simulink model "Swarm_Offline"  (Simulink 8.0)
settings: Solver=ode5  StartTime=0.0  StopTime=inf  FixedStep=sample_time  RelTol=1e-3
InitFcn:
  | sample_time=0.005;%0.004;%0.0025;%0.02;
  | sample_time_Vicon = 0.005;
  | DeltaT = 0.02;
  | g = 9.81;
  | H0 = g%0.3165;
  | Kl = 1;
  | 
  | Q6_mass = 0.73;
  | 
  | Q6_Omega_r = 1.5; %for horizon ref
  | Q6_Zeta_r = 0.5; %for horizon ref
  | Q6_Omega_r_h = 2;%for vertical ref
  | Q6_Zeta_r_h = 1; %for vertical ref
  | 
  | Q6_Omega = 1.5; %for horizon control
  | Q6_Zeta = 0.5; %for horizon control
  | Q6_Omega_h= 2; %for vertical control
  | Q6_Zeta_h = 0.7; %for vertical control
  | 
  | Q6_acc_max = 5;%horizontal max acc
  | Q6_acc_max_h = 3;%horizontal max acc
  | 
  | omega_circle = 36*pi/180;
  | omega_h = 0.1;%Ascending speed
  | PI = pi;
  | Circle_R = 2;
  | MAX_Height = -1;
  | 
  | r0=2; %desired separation distance
  | num = 3; %number of neighbors
  | 
  | load UAV1.mat
  | load UAV2.mat
  | load UAV3.mat
  | load UAV4.mat
libraries: X330_Control x22, simulink x12
(part 2 of 3)

== system Swarm_Offline/Agent 3/Swarming/swarm ==
  agent : Inport
  follower : Inport  Port=2
  2 UAV Swarm Algorithm : MATLAB Function  TreatAsAtomicUnit=on
  Constant : Constant  Value=r0
  agent cmd : Outport
  wires:
  agent/1 -> 2 UAV Swarm Algorithm/1(pos1)
  follower/1 -> 2 UAV Swarm Algorithm/2(pos2)
  2 UAV Swarm Algorithm/2(pos_cmd1) -> agent cmd/1
  Constant/1 -> 2 UAV Swarm Algorithm/3(r0)

== system Swarm_Offline/Agent 3/Swarming/swarm1 ==
  agent : Inport
  follower : Inport  Port=2
  2 UAV Swarm Algorithm : MATLAB Function  TreatAsAtomicUnit=on
  Constant : Constant  Value=r0
  agent cmd : Outport
  wires:
  Constant/1 -> 2 UAV Swarm Algorithm/3(r0)
  2 UAV Swarm Algorithm/2(pos_cmd1) -> agent cmd/1
  follower/1 -> 2 UAV Swarm Algorithm/2(pos2)
  agent/1 -> 2 UAV Swarm Algorithm/1(pos1)

== system Swarm_Offline/Agent 3/Swarming/swarm2 ==
  agent : Inport
  follower : Inport  Port=2
  2 UAV Swarm Algorithm : MATLAB Function  TreatAsAtomicUnit=on
  Constant : Constant  Value=r0
  agent cmd : Outport
  wires:
  agent/1 -> 2 UAV Swarm Algorithm/1(pos1)
  follower/1 -> 2 UAV Swarm Algorithm/2(pos2)
  2 UAV Swarm Algorithm/2(pos_cmd1) -> agent cmd/1
  Constant/1 -> 2 UAV Swarm Algorithm/3(r0)

== system Swarm_Offline/Agent 4/Swarming/swarm ==
  agent : Inport
  follower : Inport  Port=2
  2 UAV Swarm Algorithm : MATLAB Function  TreatAsAtomicUnit=on
  Constant : Constant  Value=r0
  agent cmd : Outport
  wires:
  Constant/1 -> 2 UAV Swarm Algorithm/3(r0)
  2 UAV Swarm Algorithm/2(pos_cmd1) -> agent cmd/1
  follower/1 -> 2 UAV Swarm Algorithm/2(pos2)
  agent/1 -> 2 UAV Swarm Algorithm/1(pos1)

== system Swarm_Offline/Agent 4/Swarming/swarm1 ==
  agent : Inport
  follower : Inport  Port=2
  2 UAV Swarm Algorithm : MATLAB Function  TreatAsAtomicUnit=on
  Constant : Constant  Value=r0
  agent cmd : Outport
  wires:
  agent/1 -> 2 UAV Swarm Algorithm/1(pos1)
  follower/1 -> 2 UAV Swarm Algorithm/2(pos2)
  2 UAV Swarm Algorithm/2(pos_cmd1) -> agent cmd/1
  Constant/1 -> 2 UAV Swarm Algorithm/3(r0)

== system Swarm_Offline/Agent 4/Swarming/swarm2 ==
  agent : Inport
  follower : Inport  Port=2
  2 UAV Swarm Algorithm : MATLAB Function  TreatAsAtomicUnit=on
  Constant : Constant  Value=r0
  agent cmd : Outport
  wires:
  Constant/1 -> 2 UAV Swarm Algorithm/3(r0)
  2 UAV Swarm Algorithm/2(pos_cmd1) -> agent cmd/1
  follower/1 -> 2 UAV Swarm Algorithm/2(pos2)
  agent/1 -> 2 UAV Swarm Algorithm/1(pos1)

== system Swarm_Offline/UAV 1/Trajectory Logic/UAV SF1/Airborne.traj ==
  u : Inport
  f : TriggerPort  TriggerType=function-call
      settings: CopyFcn=Stateflow.SLINSF.SimulinkMan.removeBlockPreDeleteFcn  PreDeleteFcn=Stateflow.SLINSF.SimulinkMan.unsafePredeleteFcn
  Constant : Constant  Value=0
  Enabled Subsystem1 : Subsystem  TreatAsAtomicUnit=on
  Sum : Sum  Inputs=|++
  y1 : Outport
  y2 : Outport  Port=2
  wires:
  Enabled Subsystem1/2(y) -> y2/1
  Enabled Subsystem1/1(x) -> y1/1
  Sum/1 -> Enabled Subsystem1/Enable
  u/1 -> Sum/1
  Constant/1 -> Sum/2

== system Swarm_Offline/UAV 3/Trajectory Logic/UAV SF1/Airborne.traj ==
  u : Inport
  f : TriggerPort  TriggerType=function-call
      settings: CopyFcn=Stateflow.SLINSF.SimulinkMan.removeBlockPreDeleteFcn  PreDeleteFcn=Stateflow.SLINSF.SimulinkMan.unsafePredeleteFcn
  Constant : Constant  Value=0
  Enabled Subsystem1 : Subsystem  TreatAsAtomicUnit=on
  Sum : Sum  Inputs=|++
  y1 : Outport
  y2 : Outport  Port=2
  wires:
  Enabled Subsystem1/2(y) -> y2/1
  Enabled Subsystem1/1(x) -> y1/1
  Sum/1 -> Enabled Subsystem1/Enable
  u/1 -> Sum/1
  Constant/1 -> Sum/2

== system Swarm_Offline/UAV 4/Trajectory Logic/UAV SF1/Airborne.traj ==
  u : Inport
  f : TriggerPort  TriggerType=function-call
      settings: CopyFcn=Stateflow.SLINSF.SimulinkMan.removeBlockPreDeleteFcn  PreDeleteFcn=Stateflow.SLINSF.SimulinkMan.unsafePredeleteFcn
  Constant : Constant  Value=0
  Enabled Subsystem1 : Subsystem  TreatAsAtomicUnit=on
  Sum : Sum  Inputs=|++
  y1 : Outport
  y2 : Outport  Port=2
  wires:
  Constant/1 -> Sum/2
  u/1 -> Sum/1
  Sum/1 -> Enabled Subsystem1/Enable
  Enabled Subsystem1/1(x) -> y1/1
  Enabled Subsystem1/2(y) -> y2/1

== system Swarm_Offline/UAV 5/Trajectory Logic/UAV SF1/Airborne.traj ==
  u : Inport
  f : TriggerPort  TriggerType=function-call
      settings: CopyFcn=Stateflow.SLINSF.SimulinkMan.removeBlockPreDeleteFcn  PreDeleteFcn=Stateflow.SLINSF.SimulinkMan.unsafePredeleteFcn
  Constant : Constant  Value=0
  Enabled Subsystem1 : Subsystem  TreatAsAtomicUnit=on
  Sum : Sum  Inputs=|++
  y1 : Outport
  y2 : Outport  Port=2
  wires:
  Constant/1 -> Sum/2
  u/1 -> Sum/1
  Sum/1 -> Enabled Subsystem1/Enable
  Enabled Subsystem1/1(x) -> y1/1
  Enabled Subsystem1/2(y) -> y2/1

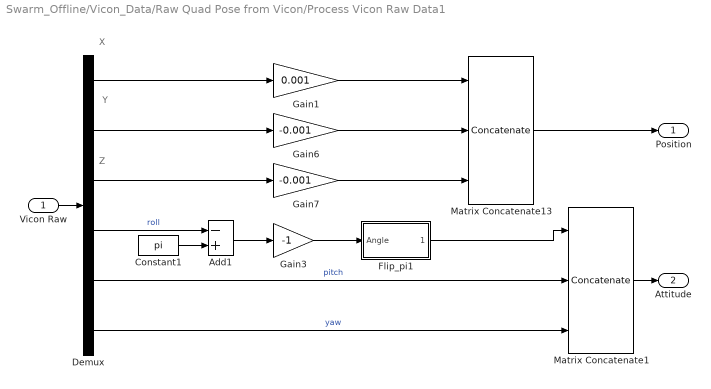
== system Swarm_Offline/Vicon_Data/Raw Quad Pose from Vicon/Process Vicon Raw Data1 ==
  note: X
  note: Y
  note: Z
  Vicon Raw : Inport
  Add1 : Sum  Inputs=-+
  Constant1 : Constant  Value=pi  OutDataTypeStr=double
  Demux : Demux  Outputs=6
  Flip_pi1 : Subsystem  mask(Flip -pi to pi){}
      mask help: Flips the inputs into the range -pi to pi
      mask Help: Flips the inputs into the range -pi to pi
      mask Display: disp('Flip_pi')
  Gain1 : Gain  Gain=0.001
  Gain3 : Gain  Gain=-1
  Gain6 : Gain  Gain=-0.001
  Gain7 : Gain  Gain=-0.001
  Matrix Concatenate1 : Concatenate  NumInputs=3  Mode=Multidimensional array
  Matrix Concatenate13 : Concatenate  NumInputs=3  Mode=Multidimensional array
  Position : Outport
  Attitude : Outport  Port=2
  wires:
  Constant1/1 -> Add1/2
  Demux/6 -> Matrix Concatenate1/3  "yaw"
  Gain1/1 -> Matrix Concatenate13/1
  Demux/1 -> Gain1/1
  Demux/2 -> Gain6/1
  Demux/3 -> Gain7/1
  Demux/4 -> Add1/1  "roll"
  Gain6/1 -> Matrix Concatenate13/2
  Gain7/1 -> Matrix Concatenate13/3
  Add1/1 -> Gain3/1
  Gain3/1 -> Flip_pi1/1(Angle)
  Demux/5 -> Matrix Concatenate1/2  "pitch"
  Flip_pi1/1(Angle_Flip) -> Matrix Concatenate1/1
  Matrix Concatenate13/1 -> Position/1
  Vicon Raw/1 -> Demux/1
  Matrix Concatenate1/1 -> Attitude/1

== system Swarm_Offline/Vicon_Data/Raw Quad Pose from Vicon/Process Vicon Raw Data2 ==
  note: Z
  note: Y
  note: X
  Vicon Raw : Inport
  Add1 : Sum  Inputs=-+
  Constant1 : Constant  Value=pi  OutDataTypeStr=double
  Demux : Demux  Outputs=6
  Flip_pi1 : Subsystem  mask(Flip -pi to pi){}
      mask help: Flips the inputs into the range -pi to pi
      mask Help: Flips the inputs into the range -pi to pi
      mask Display: disp('Flip_pi')
  Gain1 : Gain  Gain=0.001
  Gain3 : Gain  Gain=-1
  Gain6 : Gain  Gain=-0.001
  Gain7 : Gain  Gain=-0.001
  Matrix Concatenate1 : Concatenate  NumInputs=3  Mode=Multidimensional array
  Matrix Concatenate13 : Concatenate  NumInputs=3  Mode=Multidimensional array
  Position : Outport
  Attitude : Outport  Port=2
  wires:
  Matrix Concatenate1/1 -> Attitude/1
  Vicon Raw/1 -> Demux/1
  Matrix Concatenate13/1 -> Position/1
  Flip_pi1/1(Angle_Flip) -> Matrix Concatenate1/1
  Demux/5 -> Matrix Concatenate1/2  "pitch"
  Gain3/1 -> Flip_pi1/1(Angle)
  Add1/1 -> Gain3/1
  Gain7/1 -> Matrix Concatenate13/3
  Gain6/1 -> Matrix Concatenate13/2
  Demux/4 -> Add1/1  "roll"
  Demux/3 -> Gain7/1
  Demux/2 -> Gain6/1
  Demux/1 -> Gain1/1
  Gain1/1 -> Matrix Concatenate13/1
  Demux/6 -> Matrix Concatenate1/3  "yaw"
  Constant1/1 -> Add1/2

== system Swarm_Offline/Vicon_Data/Raw Quad Pose from Vicon/Process Vicon Raw Data3 ==
  note: Z
  note: Y
  note: X
  Vicon Raw : Inport
  Add1 : Sum  Inputs=-+
  Constant1 : Constant  Value=pi  OutDataTypeStr=double
  Demux : Demux  Outputs=6
  Flip_pi1 : Subsystem  mask(Flip -pi to pi){}
      mask help: Flips the inputs into the range -pi to pi
      mask Help: Flips the inputs into the range -pi to pi
      mask Display: disp('Flip_pi')
  Gain1 : Gain  Gain=0.001
  Gain3 : Gain  Gain=-1
  Gain6 : Gain  Gain=-0.001
  Gain7 : Gain  Gain=-0.001
  Matrix Concatenate1 : Concatenate  NumInputs=3  Mode=Multidimensional array
  Matrix Concatenate13 : Concatenate  NumInputs=3  Mode=Multidimensional array
  Position : Outport
  Attitude : Outport  Port=2
  wires:
  Matrix Concatenate1/1 -> Attitude/1
  Vicon Raw/1 -> Demux/1
  Matrix Concatenate13/1 -> Position/1
  Flip_pi1/1(Angle_Flip) -> Matrix Concatenate1/1
  Demux/5 -> Matrix Concatenate1/2  "pitch"
  Gain3/1 -> Flip_pi1/1(Angle)
  Add1/1 -> Gain3/1
  Gain7/1 -> Matrix Concatenate13/3
  Gain6/1 -> Matrix Concatenate13/2
  Demux/4 -> Add1/1  "roll"
  Demux/3 -> Gain7/1
  Demux/2 -> Gain6/1
  Demux/1 -> Gain1/1
  Gain1/1 -> Matrix Concatenate13/1
  Demux/6 -> Matrix Concatenate1/3  "yaw"
  Constant1/1 -> Add1/2

== system Swarm_Offline/Vicon_Data/Raw Quad Pose from Vicon/Process Vicon Raw Data4 ==
  note: X
  note: Y
  note: Z
  Vicon Raw : Inport
  Add1 : Sum  Inputs=-+
  Constant1 : Constant  Value=pi  OutDataTypeStr=double
  Demux : Demux  Outputs=6
  Flip_pi1 : Subsystem  mask(Flip -pi to pi){}
      mask help: Flips the inputs into the range -pi to pi
      mask Help: Flips the inputs into the range -pi to pi
      mask Display: disp('Flip_pi')
  Gain1 : Gain  Gain=0.001
  Gain3 : Gain  Gain=-1
  Gain6 : Gain  Gain=-0.001
  Gain7 : Gain  Gain=-0.001
  Matrix Concatenate1 : Concatenate  NumInputs=3  Mode=Multidimensional array
  Matrix Concatenate13 : Concatenate  NumInputs=3  Mode=Multidimensional array
  Position : Outport
  Attitude : Outport  Port=2
  wires:
  Constant1/1 -> Add1/2
  Demux/6 -> Matrix Concatenate1/3  "yaw"
  Gain1/1 -> Matrix Concatenate13/1
  Demux/1 -> Gain1/1
  Demux/2 -> Gain6/1
  Demux/3 -> Gain7/1
  Demux/4 -> Add1/1  "roll"
  Gain6/1 -> Matrix Concatenate13/2
  Gain7/1 -> Matrix Concatenate13/3
  Add1/1 -> Gain3/1
  Gain3/1 -> Flip_pi1/1(Angle)
  Demux/5 -> Matrix Concatenate1/2  "pitch"
  Flip_pi1/1(Angle_Flip) -> Matrix Concatenate1/1
  Matrix Concatenate13/1 -> Position/1
  Vicon Raw/1 -> Demux/1
  Matrix Concatenate1/1 -> Attitude/1

== system Swarm_Offline/Vicon_Data/Raw Quad Pose from Vicon/Process Vicon Raw Data6 ==
  note: X
  note: Y
  note: Z
  Vicon Raw : Inport
  Add1 : Sum  Inputs=-+
  Constant1 : Constant  Value=pi  OutDataTypeStr=double
  Demux : Demux  Outputs=6
  Flip_pi1 : Subsystem  mask(Flip -pi to pi){}
      mask help: Flips the inputs into the range -pi to pi
      mask Help: Flips the inputs into the range -pi to pi
      mask Display: disp('Flip_pi')
  Gain1 : Gain  Gain=0.001
  Gain3 : Gain  Gain=-1
  Gain6 : Gain  Gain=-0.001
  Gain7 : Gain  Gain=-0.001
  Matrix Concatenate1 : Concatenate  NumInputs=3  Mode=Multidimensional array
  Matrix Concatenate13 : Concatenate  NumInputs=3  Mode=Multidimensional array
  Position : Outport
  Attitude : Outport  Port=2
  wires:
  Constant1/1 -> Add1/2
  Demux/6 -> Matrix Concatenate1/3  "yaw"
  Gain1/1 -> Matrix Concatenate13/1
  Demux/1 -> Gain1/1
  Demux/2 -> Gain6/1
  Demux/3 -> Gain7/1
  Demux/4 -> Add1/1  "roll"
  Gain6/1 -> Matrix Concatenate13/2
  Gain7/1 -> Matrix Concatenate13/3
  Add1/1 -> Gain3/1
  Gain3/1 -> Flip_pi1/1(Angle)
  Demux/5 -> Matrix Concatenate1/2  "pitch"
  Flip_pi1/1(Angle_Flip) -> Matrix Concatenate1/1
  Matrix Concatenate13/1 -> Position/1
  Vicon Raw/1 -> Demux/1
  Matrix Concatenate1/1 -> Attitude/1

== system Swarm_Offline/Vicon_Data/Raw Quad Pose from Vicon/Process Vicon Raw Data7 ==
  note: Z
  note: Y
  note: X
  Vicon Raw : Inport
  Add1 : Sum  Inputs=-+
  Constant1 : Constant  Value=pi  OutDataTypeStr=double
  Demux : Demux  Outputs=6
  Flip_pi1 : Subsystem  mask(Flip -pi to pi){}
      mask help: Flips the inputs into the range -pi to pi
      mask Help: Flips the inputs into the range -pi to pi
      mask Display: disp('Flip_pi')
  Gain1 : Gain  Gain=0.001
  Gain3 : Gain  Gain=-1
  Gain6 : Gain  Gain=-0.001
  Gain7 : Gain  Gain=-0.001
  Matrix Concatenate1 : Concatenate  NumInputs=3  Mode=Multidimensional array
  Matrix Concatenate13 : Concatenate  NumInputs=3  Mode=Multidimensional array
  Position : Outport
  Attitude : Outport  Port=2
  wires:
  Matrix Concatenate1/1 -> Attitude/1
  Vicon Raw/1 -> Demux/1
  Matrix Concatenate13/1 -> Position/1
  Flip_pi1/1(Angle_Flip) -> Matrix Concatenate1/1
  Demux/5 -> Matrix Concatenate1/2  "pitch"
  Gain3/1 -> Flip_pi1/1(Angle)
  Add1/1 -> Gain3/1
  Gain7/1 -> Matrix Concatenate13/3
  Gain6/1 -> Matrix Concatenate13/2
  Demux/4 -> Add1/1  "roll"
  Demux/3 -> Gain7/1
  Demux/2 -> Gain6/1
  Demux/1 -> Gain1/1
  Gain1/1 -> Matrix Concatenate13/1
  Demux/6 -> Matrix Concatenate1/3  "yaw"
  Constant1/1 -> Add1/2

== system Swarm_Offline/UAV 1/Trajectory Logic/UAV SF1/Airborne.traj/Enabled Subsystem1 ==
  Enable : EnablePort
  From Workspace : FromWorkspace  VariableName=UAV1  Interpolate=off  OutputAfterFinalValue=Holding final value
  Selector1 : Selector  InputPortWidth=2  IndexOptions=Index vector (dialog)  Indices=[2]  OutputSizes=1
  Selector6 : Selector  InputPortWidth=2  IndexOptions=Index vector (dialog)  Indices=[1]  OutputSizes=1
  x : Outport
  y : Outport  Port=2
  z : Outport  Port=3
  Psi : Outport  Port=4
  wires:
  Selector1/1 -> y/1
  Selector6/1 -> x/1
  From Workspace/1 -> Selector6/1, Selector1/1

== system Swarm_Offline/UAV 3/Trajectory Logic/UAV SF1/Airborne.traj/Enabled Subsystem1 ==
  Enable : EnablePort
  From Workspace : FromWorkspace  VariableName=UAV2  Interpolate=off  OutputAfterFinalValue=Holding final value
  Selector1 : Selector  InputPortWidth=2  IndexOptions=Index vector (dialog)  Indices=[1]  OutputSizes=1
  Selector6 : Selector  InputPortWidth=2  IndexOptions=Index vector (dialog)  Indices=[1]  OutputSizes=1
  x : Outport
  y : Outport  Port=2
  z : Outport  Port=3
  Psi : Outport  Port=4
  wires:
  Selector6/1 -> y/1
  Selector1/1 -> x/1
  From Workspace/1 -> Selector1/1, Selector6/1

== system Swarm_Offline/UAV 4/Trajectory Logic/UAV SF1/Airborne.traj/Enabled Subsystem1 ==
  Enable : EnablePort
  From Workspace : FromWorkspace  VariableName=UAV3  Interpolate=off  OutputAfterFinalValue=Holding final value
  Selector1 : Selector  InputPortWidth=2  IndexOptions=Index vector (dialog)  Indices=[1]  OutputSizes=1
  Selector6 : Selector  InputPortWidth=2  IndexOptions=Index vector (dialog)  Indices=[1]  OutputSizes=1
  x : Outport
  y : Outport  Port=2
  z : Outport  Port=3
  psi : Outport  Port=4
  wires:
  From Workspace/1 -> Selector1/1, Selector6/1
  Selector1/1 -> x/1
  Selector6/1 -> y/1

== system Swarm_Offline/UAV 5/Trajectory Logic/UAV SF1/Airborne.traj/Enabled Subsystem1 ==
  Enable : EnablePort
  From Workspace : FromWorkspace  VariableName=UAV4  Interpolate=off  OutputAfterFinalValue=Holding final value
  Selector1 : Selector  InputPortWidth=2  IndexOptions=Index vector (dialog)  Indices=[1]  OutputSizes=1
  Selector6 : Selector  InputPortWidth=2  IndexOptions=Index vector (dialog)  Indices=[1]  OutputSizes=1
  x : Outport
  y : Outport  Port=2
  z : Outport  Port=3
  Psi : Outport  Port=4
  wires:
  From Workspace/1 -> Selector6/1, Selector1/1
  Selector1/1 -> x/1
  Selector6/1 -> y/1

== system Swarm_Offline/Vicon_Data/Raw Quad Pose from Vicon/Process Vicon Raw Data1/Flip_pi1 ==
  Angle : Inport
  Add : Sum  Inputs=-+
  Compare To Constant1 : simulink/Logic and Bit Operations/Compare To Constant  relop=>  const=pi  OutDataTypeStr=uint8  ZeroCross=off
  Constant : Constant  Value=2*pi
  Data Type Duplicate : DataTypeDuplicate
  Flip_0_to_2pi : Subsystem  mask(Flip zero to 2pi){}
      mask help: Flips the inputs into the range zero to +2pi
      mask Help: Flips the inputs into the range zero to +2pi
      mask Display: disp('Flip_0_2pi')
  Switch : Switch  Criteria=u2 ~= 0
  Angle_Flip : Outport
  wires:
  Switch/1 -> Data Type Duplicate/1, Angle_Flip/1
  Add/1 -> Switch/1
  Constant/1 -> Add/1
  Compare To Constant1/1 -> Switch/2
  Flip_0_to_2pi/1(Angle_Flip) -> Add/2, Compare To Constant1/1, Switch/3
  Angle/1 -> Data Type Duplicate/2, Flip_0_to_2pi/1(Angle)

== system Swarm_Offline/Vicon_Data/Raw Quad Pose from Vicon/Process Vicon Raw Data2/Flip_pi1 ==
  Angle : Inport
  Add : Sum  Inputs=-+
  Compare To Constant1 : simulink/Logic and Bit Operations/Compare To Constant  relop=>  const=pi  OutDataTypeStr=uint8  ZeroCross=off
  Constant : Constant  Value=2*pi
  Data Type Duplicate : DataTypeDuplicate
  Flip_0_to_2pi : Subsystem  mask(Flip zero to 2pi){}
      mask help: Flips the inputs into the range zero to +2pi
      mask Help: Flips the inputs into the range zero to +2pi
      mask Display: disp('Flip_0_2pi')
  Switch : Switch  Criteria=u2 ~= 0
  Angle_Flip : Outport
  wires:
  Angle/1 -> Flip_0_to_2pi/1(Angle), Data Type Duplicate/2
  Flip_0_to_2pi/1(Angle_Flip) -> Switch/3, Compare To Constant1/1, Add/2
  Compare To Constant1/1 -> Switch/2
  Constant/1 -> Add/1
  Add/1 -> Switch/1
  Switch/1 -> Angle_Flip/1, Data Type Duplicate/1

== system Swarm_Offline/Vicon_Data/Raw Quad Pose from Vicon/Process Vicon Raw Data3/Flip_pi1 ==
  Angle : Inport
  Add : Sum  Inputs=-+
  Compare To Constant1 : simulink/Logic and Bit Operations/Compare To Constant  relop=>  const=pi  OutDataTypeStr=uint8  ZeroCross=off
  Constant : Constant  Value=2*pi
  Data Type Duplicate : DataTypeDuplicate
  Flip_0_to_2pi : Subsystem  mask(Flip zero to 2pi){}
      mask help: Flips the inputs into the range zero to +2pi
      mask Help: Flips the inputs into the range zero to +2pi
      mask Display: disp('Flip_0_2pi')
  Switch : Switch  Criteria=u2 ~= 0
  Angle_Flip : Outport
  wires:
  Angle/1 -> Flip_0_to_2pi/1(Angle), Data Type Duplicate/2
  Flip_0_to_2pi/1(Angle_Flip) -> Switch/3, Compare To Constant1/1, Add/2
  Compare To Constant1/1 -> Switch/2
  Constant/1 -> Add/1
  Add/1 -> Switch/1
  Switch/1 -> Angle_Flip/1, Data Type Duplicate/1

== system Swarm_Offline/Vicon_Data/Raw Quad Pose from Vicon/Process Vicon Raw Data4/Flip_pi1 ==
  Angle : Inport
  Add : Sum  Inputs=-+
  Compare To Constant1 : simulink/Logic and Bit Operations/Compare To Constant  relop=>  const=pi  OutDataTypeStr=uint8  ZeroCross=off
  Constant : Constant  Value=2*pi
  Data Type Duplicate : DataTypeDuplicate
  Flip_0_to_2pi : Subsystem  mask(Flip zero to 2pi){}
      mask help: Flips the inputs into the range zero to +2pi
      mask Help: Flips the inputs into the range zero to +2pi
      mask Display: disp('Flip_0_2pi')
  Switch : Switch  Criteria=u2 ~= 0
  Angle_Flip : Outport
  wires:
  Switch/1 -> Data Type Duplicate/1, Angle_Flip/1
  Add/1 -> Switch/1
  Constant/1 -> Add/1
  Compare To Constant1/1 -> Switch/2
  Flip_0_to_2pi/1(Angle_Flip) -> Add/2, Compare To Constant1/1, Switch/3
  Angle/1 -> Data Type Duplicate/2, Flip_0_to_2pi/1(Angle)

== system Swarm_Offline/Vicon_Data/Raw Quad Pose from Vicon/Process Vicon Raw Data6/Flip_pi1 ==
  Angle : Inport
  Add : Sum  Inputs=-+
  Compare To Constant1 : simulink/Logic and Bit Operations/Compare To Constant  relop=>  const=pi  OutDataTypeStr=uint8  ZeroCross=off
  Constant : Constant  Value=2*pi
  Data Type Duplicate : DataTypeDuplicate
  Flip_0_to_2pi : Subsystem  mask(Flip zero to 2pi){}
      mask help: Flips the inputs into the range zero to +2pi
      mask Help: Flips the inputs into the range zero to +2pi
      mask Display: disp('Flip_0_2pi')
  Switch : Switch  Criteria=u2 ~= 0
  Angle_Flip : Outport
  wires:
  Switch/1 -> Data Type Duplicate/1, Angle_Flip/1
  Add/1 -> Switch/1
  Constant/1 -> Add/1
  Compare To Constant1/1 -> Switch/2
  Flip_0_to_2pi/1(Angle_Flip) -> Add/2, Compare To Constant1/1, Switch/3
  Angle/1 -> Data Type Duplicate/2, Flip_0_to_2pi/1(Angle)

== system Swarm_Offline/Vicon_Data/Raw Quad Pose from Vicon/Process Vicon Raw Data7/Flip_pi1 ==
  Angle : Inport
  Add : Sum  Inputs=-+
  Compare To Constant1 : simulink/Logic and Bit Operations/Compare To Constant  relop=>  const=pi  OutDataTypeStr=uint8  ZeroCross=off
  Constant : Constant  Value=2*pi
  Data Type Duplicate : DataTypeDuplicate
  Flip_0_to_2pi : Subsystem  mask(Flip zero to 2pi){}
      mask help: Flips the inputs into the range zero to +2pi
      mask Help: Flips the inputs into the range zero to +2pi
      mask Display: disp('Flip_0_2pi')
  Switch : Switch  Criteria=u2 ~= 0
  Angle_Flip : Outport
  wires:
  Angle/1 -> Flip_0_to_2pi/1(Angle), Data Type Duplicate/2
  Flip_0_to_2pi/1(Angle_Flip) -> Switch/3, Compare To Constant1/1, Add/2
  Compare To Constant1/1 -> Switch/2
  Constant/1 -> Add/1
  Add/1 -> Switch/1
  Switch/1 -> Angle_Flip/1, Data Type Duplicate/1

== system Swarm_Offline/Vicon_Data/Raw Quad Pose from Vicon/Process Vicon Raw Data1/Flip_pi1/Flip_0_to_2pi ==
  Angle : Inport
  Add : Sum
  Compare To Constant1 : simulink/Logic and Bit Operations/Compare To Constant  relop=<  const=0  OutDataTypeStr=uint8  ZeroCross=off
  Constant : Constant  Value=2*pi
  Data Type Duplicate : DataTypeDuplicate
  Flip_2pi : Subsystem  mask(Flip -2pi to 2pi){}
      mask help: Flips the inputs into the range -2pi to +2pi
      mask Help: Flips the inputs into the range -2pi to +2pi
      mask Display: disp('Flip_2pi')
  Switch : Switch  Criteria=u2 ~= 0
  Angle_Flip : Outport
  wires:
  Switch/1 -> Data Type Duplicate/1, Angle_Flip/1
  Angle/1 -> Data Type Duplicate/2, Flip_2pi/1(Angle)
  Add/1 -> Switch/1
  Constant/1 -> Add/1
  Compare To Constant1/1 -> Switch/2
  Flip_2pi/1(Angle_Flip) -> Switch/3, Add/2, Compare To Constant1/1

== system Swarm_Offline/Vicon_Data/Raw Quad Pose from Vicon/Process Vicon Raw Data2/Flip_pi1/Flip_0_to_2pi ==
  Angle : Inport
  Add : Sum
  Compare To Constant1 : simulink/Logic and Bit Operations/Compare To Constant  relop=<  const=0  OutDataTypeStr=uint8  ZeroCross=off
  Constant : Constant  Value=2*pi
  Data Type Duplicate : DataTypeDuplicate
  Flip_2pi : Subsystem  mask(Flip -2pi to 2pi){}
      mask help: Flips the inputs into the range -2pi to +2pi
      mask Help: Flips the inputs into the range -2pi to +2pi
      mask Display: disp('Flip_2pi')
  Switch : Switch  Criteria=u2 ~= 0
  Angle_Flip : Outport
  wires:
  Flip_2pi/1(Angle_Flip) -> Compare To Constant1/1, Add/2, Switch/3
  Compare To Constant1/1 -> Switch/2
  Constant/1 -> Add/1
  Add/1 -> Switch/1
  Angle/1 -> Flip_2pi/1(Angle), Data Type Duplicate/2
  Switch/1 -> Angle_Flip/1, Data Type Duplicate/1

== system Swarm_Offline/Vicon_Data/Raw Quad Pose from Vicon/Process Vicon Raw Data3/Flip_pi1/Flip_0_to_2pi ==
  Angle : Inport
  Add : Sum
  Compare To Constant1 : simulink/Logic and Bit Operations/Compare To Constant  relop=<  const=0  OutDataTypeStr=uint8  ZeroCross=off
  Constant : Constant  Value=2*pi
  Data Type Duplicate : DataTypeDuplicate
  Flip_2pi : Subsystem  mask(Flip -2pi to 2pi){}
      mask help: Flips the inputs into the range -2pi to +2pi
      mask Help: Flips the inputs into the range -2pi to +2pi
      mask Display: disp('Flip_2pi')
  Switch : Switch  Criteria=u2 ~= 0
  Angle_Flip : Outport
  wires:
  Flip_2pi/1(Angle_Flip) -> Compare To Constant1/1, Add/2, Switch/3
  Compare To Constant1/1 -> Switch/2
  Constant/1 -> Add/1
  Add/1 -> Switch/1
  Angle/1 -> Flip_2pi/1(Angle), Data Type Duplicate/2
  Switch/1 -> Angle_Flip/1, Data Type Duplicate/1

== system Swarm_Offline/Vicon_Data/Raw Quad Pose from Vicon/Process Vicon Raw Data4/Flip_pi1/Flip_0_to_2pi ==
  Angle : Inport
  Add : Sum
  Compare To Constant1 : simulink/Logic and Bit Operations/Compare To Constant  relop=<  const=0  OutDataTypeStr=uint8  ZeroCross=off
  Constant : Constant  Value=2*pi
  Data Type Duplicate : DataTypeDuplicate
  Flip_2pi : Subsystem  mask(Flip -2pi to 2pi){}
      mask help: Flips the inputs into the range -2pi to +2pi
      mask Help: Flips the inputs into the range -2pi to +2pi
      mask Display: disp('Flip_2pi')
  Switch : Switch  Criteria=u2 ~= 0
  Angle_Flip : Outport
  wires:
  Switch/1 -> Data Type Duplicate/1, Angle_Flip/1
  Angle/1 -> Data Type Duplicate/2, Flip_2pi/1(Angle)
  Add/1 -> Switch/1
  Constant/1 -> Add/1
  Compare To Constant1/1 -> Switch/2
  Flip_2pi/1(Angle_Flip) -> Switch/3, Add/2, Compare To Constant1/1

== system Swarm_Offline/Vicon_Data/Raw Quad Pose from Vicon/Process Vicon Raw Data6/Flip_pi1/Flip_0_to_2pi ==
  Angle : Inport
  Add : Sum
  Compare To Constant1 : simulink/Logic and Bit Operations/Compare To Constant  relop=<  const=0  OutDataTypeStr=uint8  ZeroCross=off
  Constant : Constant  Value=2*pi
  Data Type Duplicate : DataTypeDuplicate
  Flip_2pi : Subsystem  mask(Flip -2pi to 2pi){}
      mask help: Flips the inputs into the range -2pi to +2pi
      mask Help: Flips the inputs into the range -2pi to +2pi
      mask Display: disp('Flip_2pi')
  Switch : Switch  Criteria=u2 ~= 0
  Angle_Flip : Outport
  wires:
  Switch/1 -> Data Type Duplicate/1, Angle_Flip/1
  Angle/1 -> Data Type Duplicate/2, Flip_2pi/1(Angle)
  Add/1 -> Switch/1
  Constant/1 -> Add/1
  Compare To Constant1/1 -> Switch/2
  Flip_2pi/1(Angle_Flip) -> Switch/3, Add/2, Compare To Constant1/1

== system Swarm_Offline/Vicon_Data/Raw Quad Pose from Vicon/Process Vicon Raw Data7/Flip_pi1/Flip_0_to_2pi ==
  Angle : Inport
  Add : Sum
  Compare To Constant1 : simulink/Logic and Bit Operations/Compare To Constant  relop=<  const=0  OutDataTypeStr=uint8  ZeroCross=off
  Constant : Constant  Value=2*pi
  Data Type Duplicate : DataTypeDuplicate
  Flip_2pi : Subsystem  mask(Flip -2pi to 2pi){}
      mask help: Flips the inputs into the range -2pi to +2pi
      mask Help: Flips the inputs into the range -2pi to +2pi
      mask Display: disp('Flip_2pi')
  Switch : Switch  Criteria=u2 ~= 0
  Angle_Flip : Outport
  wires:
  Flip_2pi/1(Angle_Flip) -> Compare To Constant1/1, Add/2, Switch/3
  Compare To Constant1/1 -> Switch/2
  Constant/1 -> Add/1
  Add/1 -> Switch/1
  Angle/1 -> Flip_2pi/1(Angle), Data Type Duplicate/2
  Switch/1 -> Angle_Flip/1, Data Type Duplicate/1

== system Swarm_Offline/Vicon_Data/Raw Quad Pose from Vicon/Process Vicon Raw Data1/Flip_pi1/Flip_0_to_2pi/Flip_2pi ==
  Angle : Inport
  Bias : Bias  Bias=-2*pi
  Constant : Constant  Value=2*pi
  Data Type Duplicate : DataTypeDuplicate
  Modulo : Math  Operator=mod  SaturateOnIntegerOverflow=on
  Sign1 : Signum
  Switch : Switch
  Angle_Flip : Outport
  wires:
  Switch/1 -> Data Type Duplicate/2, Angle_Flip/1
  Bias/1 -> Switch/3
  Sign1/1 -> Switch/2
  Modulo/1 -> Switch/1, Bias/1
  Constant/1 -> Modulo/2
  Angle/1 -> Data Type Duplicate/1, Sign1/1, Modulo/1

== system Swarm_Offline/Vicon_Data/Raw Quad Pose from Vicon/Process Vicon Raw Data2/Flip_pi1/Flip_0_to_2pi/Flip_2pi ==
  Angle : Inport
  Bias : Bias  Bias=-2*pi
  Constant : Constant  Value=2*pi
  Data Type Duplicate : DataTypeDuplicate
  Modulo : Math  Operator=mod  SaturateOnIntegerOverflow=on
  Sign1 : Signum
  Switch : Switch
  Angle_Flip : Outport
  wires:
  Angle/1 -> Modulo/1, Sign1/1, Data Type Duplicate/1
  Constant/1 -> Modulo/2
  Modulo/1 -> Bias/1, Switch/1
  Sign1/1 -> Switch/2
  Bias/1 -> Switch/3
  Switch/1 -> Angle_Flip/1, Data Type Duplicate/2

== system Swarm_Offline/Vicon_Data/Raw Quad Pose from Vicon/Process Vicon Raw Data3/Flip_pi1/Flip_0_to_2pi/Flip_2pi ==
  Angle : Inport
  Bias : Bias  Bias=-2*pi
  Constant : Constant  Value=2*pi
  Data Type Duplicate : DataTypeDuplicate
  Modulo : Math  Operator=mod  SaturateOnIntegerOverflow=on
  Sign1 : Signum
  Switch : Switch
  Angle_Flip : Outport
  wires:
  Angle/1 -> Modulo/1, Sign1/1, Data Type Duplicate/1
  Constant/1 -> Modulo/2
  Modulo/1 -> Bias/1, Switch/1
  Sign1/1 -> Switch/2
  Bias/1 -> Switch/3
  Switch/1 -> Angle_Flip/1, Data Type Duplicate/2

== system Swarm_Offline/Vicon_Data/Raw Quad Pose from Vicon/Process Vicon Raw Data4/Flip_pi1/Flip_0_to_2pi/Flip_2pi ==
  Angle : Inport
  Bias : Bias  Bias=-2*pi
  Constant : Constant  Value=2*pi
  Data Type Duplicate : DataTypeDuplicate
  Modulo : Math  Operator=mod  SaturateOnIntegerOverflow=on
  Sign1 : Signum
  Switch : Switch
  Angle_Flip : Outport
  wires:
  Switch/1 -> Data Type Duplicate/2, Angle_Flip/1
  Bias/1 -> Switch/3
  Sign1/1 -> Switch/2
  Modulo/1 -> Switch/1, Bias/1
  Constant/1 -> Modulo/2
  Angle/1 -> Data Type Duplicate/1, Sign1/1, Modulo/1

== system Swarm_Offline/Vicon_Data/Raw Quad Pose from Vicon/Process Vicon Raw Data6/Flip_pi1/Flip_0_to_2pi/Flip_2pi ==
  Angle : Inport
  Bias : Bias  Bias=-2*pi
  Constant : Constant  Value=2*pi
  Data Type Duplicate : DataTypeDuplicate
  Modulo : Math  Operator=mod  SaturateOnIntegerOverflow=on
  Sign1 : Signum
  Switch : Switch
  Angle_Flip : Outport
  wires:
  Switch/1 -> Data Type Duplicate/2, Angle_Flip/1
  Bias/1 -> Switch/3
  Sign1/1 -> Switch/2
  Modulo/1 -> Switch/1, Bias/1
  Constant/1 -> Modulo/2
  Angle/1 -> Data Type Duplicate/1, Sign1/1, Modulo/1

== system Swarm_Offline/Vicon_Data/Raw Quad Pose from Vicon/Process Vicon Raw Data7/Flip_pi1/Flip_0_to_2pi/Flip_2pi ==
  Angle : Inport
  Bias : Bias  Bias=-2*pi
  Constant : Constant  Value=2*pi
  Data Type Duplicate : DataTypeDuplicate
  Modulo : Math  Operator=mod  SaturateOnIntegerOverflow=on
  Sign1 : Signum
  Switch : Switch
  Angle_Flip : Outport
  wires:
  Angle/1 -> Modulo/1, Sign1/1, Data Type Duplicate/1
  Constant/1 -> Modulo/2
  Modulo/1 -> Bias/1, Switch/1
  Sign1/1 -> Switch/2
  Bias/1 -> Switch/3
  Switch/1 -> Angle_Flip/1, Data Type Duplicate/2

== matlab function Agent 1/Swarming/swarm/2 UAV Swarm Algorithm ==
  data: w output double; pos1 input double; pos_cmd1 output double; pos2 input double; r0 input double
function [w,pos_cmd1] = fcn(pos1,pos2,r0)

% Swarm algorithm for Vicon environment. 
% Heading concensus is not considered, only positions. 
% Hence, only the inter-agent potential in terms of separation distance is
% taken into consideration. 
%
% Adapted from func_swarm_2UAV_2D_decentralized.m

% 25 Apr 2011

%r0 = 2;   % desired separation

delta = pos2(1:2) - pos1(1:2);
b   = 0.1;
pos_cmd1 = zeros(4,1);
w = 0;

r = norm(delta) - r0;                 % relative distance

if abs(r) < b
    w = 0;
else if r > b
    w = (2/(1+exp(-4*(r-b)))-1)*1;          % potential, max value at r=1.5m
    else if r < -b
            w = (2/(1+exp(-4*(r+b)))-1)*1;
        end
    end
end                                       % scaled by 1.0

theta = atan2(delta(2),delta(1));

pos_cmd1(1) = w*cos(theta);
pos_cmd1(2) = w*sin(theta);

% vel_cmd2(1) = -w*cos(theta);  
% vel_cmd2(2) = -w*sin(theta);

== stateflow chart UAV 3/Trajectory Logic/UAV SF1 ==
  state Landing
    state Decsending
      en:PosDesired = Pos;
      du:PosDesired[2] = (0 - PosDesired[2])*1*DeltaT + PosDesired[2] ;
    state CutThrottle
      du:HoverThrottle = (0.01 - HoverThrottle)*2*DeltaT + HoverThrottle ;
    (default) -> Decsending
    Decsending -> CutThrottle : [Pos[2] > -0.15]
  state Airborne
    state TakeOff
      du:HoverThrottle = (H0 - HoverThrottle)*2*DeltaT + HoverThrottle ;
    state Hover
      en: PosDesired[2] = -1;
    state [y1,y2] = traj(u) [function]
    state Trajectory
      state Swarm
        du:
        [PosDesired[0], PosDesired[1]] = traj(1);
        PosDesired[2] = PerchPos[2];
      state Hover
        en:
        PosDesired[0] = -2.5;
        PosDesired[1] = 3.75;
        PosDesired[2] = -1;
      state Hover1
        en:
        PosDesired = Pos;
      (default) -> Airborne.Trajectory.Hover
      Airborne.Trajectory.Hover -> Swarm : after(5,sec)
      Swarm -> Hover1 : after(15,sec)
    (default) -> TakeOff : {PosDesired = Pos;  PosDesired[2] = -1;}
    TakeOff -> Airborne.Hover : after(5,sec)
        | {PosDesired = Pos;}
    Trajectory -> Airborne.Hover : [RC[5] < 0]
        | {PosDesired = Pos;}
    Airborne.Hover -> Trajectory : [RC[5] > 0]
  Landing -> Airborne : [RC[6] > 0.5]
  Airborne -> Landing : [RC[6] < -0.5]
  (default) -> Landing : {HoverThrottle=0.01;}
  data: u function_input double; y1 function_output double; y2 function_output double; PosDesired output double size=4; HoverThrottle output double size=1; Mode output uint8 size=3; RC input double size=8; Pos input double size=4; PerchPos input double size=4; DeltaT parameter double size=1; H0 parameter double size=1; Kl parameter double size=1; VelCmd local double size=2 =0; line_count local int8 size=1 =0; triangle_count local int8 size=1 =0; T_circle local double size=1; omega_circle parameter double size=1; PI parameter double size=1; omega_h parameter double size=1; Circle_R parameter double size=1; MAX_Height parameter double size=1

== stateflow chart UAV 4/Trajectory Logic/UAV SF1 ==
  state Landing
    state Decsending
      en:PosDesired = Pos;
      du:PosDesired[2] = (0 - PosDesired[2])*1*DeltaT + PosDesired[2] ;
    state CutThrottle
      du:HoverThrottle = (0.01 - HoverThrottle)*2*DeltaT + HoverThrottle ;
    (default) -> Decsending
    Decsending -> CutThrottle : [Pos[2] > -0.15]
  state Airborne
    state TakeOff
      du:HoverThrottle = (H0 - HoverThrottle)*2*DeltaT + HoverThrottle ;
    state Hover
      en: PosDesired[2] = -1;
    state [y1,y2] = traj(u) [function]
    state Trajectory
      state Hover1
        en:
        PosDesired = Pos;
      state Swarm
        du:
        [PosDesired[0], PosDesired[1]] = traj(1);
        PosDesired[2] = PerchPos[2];
      state Hover
        en:
        PosDesired[0] = -1.75;
        PosDesired[1] = 1.25;
        PosDesired[2] = -1;
      (default) -> Airborne.Trajectory.Hover
      Airborne.Trajectory.Hover -> Swarm : after(5,sec)
      Swarm -> Hover1 : after(15,sec)
    (default) -> TakeOff : {PosDesired = Pos;  PosDesired[2] = -1;}
    TakeOff -> Airborne.Hover : after(5,sec)
        | {PosDesired = Pos;}
    Airborne.Hover -> Trajectory : [RC[5] > 0]
    Trajectory -> Airborne.Hover : [RC[5] < 0]
        | {PosDesired = Pos;}
  Landing -> Airborne : [RC[6] > 0.5]
  Airborne -> Landing : [RC[6] < -0.5]
  (default) -> Landing : {HoverThrottle=0.01;}
  data: u function_input double; y1 function_output double; y2 function_output double; PosDesired output double size=4; HoverThrottle output double size=1; Mode output uint8 size=3; RC input double size=8; Pos input double size=4; PerchPos input double size=4; DeltaT parameter double size=1; H0 parameter double size=1; Kl parameter double size=1; VelCmd local double size=2 =0; line_count local int8 size=1 =0; triangle_count local int8 size=1 =0; T_circle local double size=1; omega_circle parameter double size=1; PI parameter double size=1; omega_h parameter double size=1; Circle_R parameter double size=1; MAX_Height parameter double size=1

== stateflow chart UAV 5/Trajectory Logic/UAV SF1 ==
  state Landing
    state Decsending
      en:PosDesired = Pos;
      du:PosDesired[2] = (0 - PosDesired[2])*1*DeltaT + PosDesired[2] ;
    state CutThrottle
      du:HoverThrottle = (0.01 - HoverThrottle)*2*DeltaT + HoverThrottle ;
    (default) -> Decsending
    Decsending -> CutThrottle : [Pos[2] > -0.15]
  state Airborne
    state TakeOff
      du:HoverThrottle = (H0 - HoverThrottle)*2*DeltaT + HoverThrottle ;
    state Hover
      en: PosDesired[2] = -1;
    state [y1,y2] = traj(u) [function]
    state Trajectory
      state Hover1
        en:
        PosDesired = Pos;
      state Swarm
        du:
        [PosDesired[0], PosDesired[1]] = traj(1);
        PosDesired[2] = PerchPos[2];
      state Hover
        en:
        PosDesired[0] = -2;
        PosDesired[1] = 0.75;
        PosDesired[2] = -1;
      (default) -> Airborne.Trajectory.Hover
      Airborne.Trajectory.Hover -> Swarm : after(5,sec)
      Swarm -> Hover1 : after(15,sec)
    (default) -> TakeOff : {PosDesired = Pos;  PosDesired[2] = -1;}
    TakeOff -> Airborne.Hover : after(5,sec)
        | {PosDesired = Pos;}
    Trajectory -> Airborne.Hover : [RC[5] < 0]
        | {PosDesired = Pos;}
    Airborne.Hover -> Trajectory : [RC[5] > 0]
  Landing -> Airborne : [RC[6] > 0.5]
  Airborne -> Landing : [RC[6] < -0.5]
  (default) -> Landing : {HoverThrottle=0.01;}
  data: u function_input double; y1 function_output double; y2 function_output double; PosDesired output double size=4; HoverThrottle output double size=1; Mode output uint8 size=3; RC input double size=8; Pos input double size=4; PerchPos input double size=4; DeltaT parameter double size=1; H0 parameter double size=1; Kl parameter double size=1; VelCmd local double size=2 =0; line_count local int8 size=1 =0; triangle_count local int8 size=1 =0; T_circle local double size=1; omega_circle parameter double size=1; PI parameter double size=1; omega_h parameter double size=1; Circle_R parameter double size=1; MAX_Height parameter double size=1

== matlab function Agent 1/Swarming/swarm1/2 UAV Swarm Algorithm ==
  data: w output double; pos1 input double; pos_cmd1 output double; pos2 input double; r0 input double
function [w,pos_cmd1] = fcn(pos1,pos2,r0)

% Swarm algorithm for Vicon environment. 
% Heading concensus is not considered, only positions. 
% Hence, only the inter-agent potential in terms of separation distance is
% taken into consideration. 
%
% Adapted from func_swarm_2UAV_2D_decentralized.m

% 25 Apr 2011

%r0 = 2;   % desired separation

delta = pos2(1:2) - pos1(1:2);
b   = 0.1;
pos_cmd1 = zeros(4,1);
w = 0;

r = norm(delta) - r0;                 % relative distance

if abs(r) < b
    w = 0;
else if r > b
    w = (2/(1+exp(-4*(r-b)))-1)*1;          % potential, max value at r=1.5m
    else if r < -b
            w = (2/(1+exp(-4*(r+b)))-1)*1;
        end
    end
end                                       % scaled by 1.0

theta = atan2(delta(2),delta(1));

pos_cmd1(1) = w*cos(theta);
pos_cmd1(2) = w*sin(theta);

% vel_cmd2(1) = -w*cos(theta);  
% vel_cmd2(2) = -w*sin(theta);

== matlab function Agent 2/Swarming/swarm/2 UAV Swarm Algorithm ==
  data: w output double; pos1 input double; pos_cmd1 output double; pos2 input double; r0 input double
function [w,pos_cmd1] = fcn(pos1,pos2,r0)

% Swarm algorithm for Vicon environment. 
% Heading concensus is not considered, only positions. 
% Hence, only the inter-agent potential in terms of separation distance is
% taken into consideration. 
%
% Adapted from func_swarm_2UAV_2D_decentralized.m

% 25 Apr 2011

%r0 = 2;   % desired separation

delta = pos2(1:2) - pos1(1:2);
b   = 0.1;
pos_cmd1 = zeros(4,1);
w = 0;

r = norm(delta) - r0;                 % relative distance

if abs(r) < b
    w = 0;
else if r > b
    w = (2/(1+exp(-4*(r-b)))-1)*1;          % potential, max value at r=1.5m
    else if r < -b
            w = (2/(1+exp(-4*(r+b)))-1)*1;
        end
    end
end                                       % scaled by 1.0

theta = atan2(delta(2),delta(1));

pos_cmd1(1) = w*cos(theta);
pos_cmd1(2) = w*sin(theta);

% vel_cmd2(1) = -w*cos(theta);  
% vel_cmd2(2) = -w*sin(theta);

== stateflow chart UAV 1/Trajectory Logic/UAV SF1 ==
  state Landing
    state Decsending
      en:PosDesired = Pos;
      du:PosDesired[2] = (0 - PosDesired[2])*1*DeltaT + PosDesired[2] ;
    state CutThrottle
      du:HoverThrottle = (0.01 - HoverThrottle)*2*DeltaT + HoverThrottle ;
    (default) -> Decsending
    Decsending -> CutThrottle : [Pos[2] > -0.15]
  state Airborne
    state TakeOff
      du:HoverThrottle = (H0 - HoverThrottle)*2*DeltaT + HoverThrottle ;
    state Hover
      en: PosDesired[2] = -1;
    state [y1,y2] = traj(u) [function]
    state Trajectory
      state Swarm
        du:
        [PosDesired[0], PosDesired[1]] = traj(1);
        PosDesired[2] = max(MAX_Height ,-1 - T_circle*omega_h);
      state Hover
        en:
        PosDesired[0] = -2.25;
        PosDesired[1] = 0.75;
        PosDesired[2] = -1;
      state Hover1
        en:
        PosDesired = Pos;
      (default) -> Airborne.Trajectory.Hover
      Airborne.Trajectory.Hover -> Swarm : after(5,sec)
          | {T_circle = 0.0;}
      Swarm -> Hover1 : after(15,sec)
    (default) -> TakeOff : {PosDesired = Pos;  PosDesired[2] = -1;}
    TakeOff -> Airborne.Hover : after(5,sec)
        | {PosDesired = Pos;}
    Trajectory -> Airborne.Hover : [RC[5] < 0]
        | {PosDesired = Pos;}
    Airborne.Hover -> Trajectory : [RC[5] > 0]
  Landing -> Airborne : [RC[6] > 0.5]
  Airborne -> Landing : [RC[6] < -0.5]
  (default) -> Landing : {HoverThrottle=0.01;}
  data: u function_input double; y1 function_output double; y2 function_output double; PosDesired output double size=4; HoverThrottle output double size=1; Mode output uint8 size=3; RC input double size=8; Pos input double size=4; PerchPos input double size=4; DeltaT parameter double size=1; H0 parameter double size=1; Kl parameter double size=1; VelCmd local double size=2 =0; line_count local int8 size=1 =0; triangle_count local int8 size=1 =0; T_circle local double size=1; omega_circle parameter double size=1; PI parameter double size=1; omega_h parameter double size=1; Circle_R parameter double size=1; MAX_Height parameter double size=1

== matlab function Agent 1/Swarming/swarm2/2 UAV Swarm Algorithm ==
  data: w output double; pos1 input double; pos_cmd1 output double; pos2 input double; r0 input double
function [w,pos_cmd1] = fcn(pos1,pos2,r0)

% Swarm algorithm for Vicon environment. 
% Heading concensus is not considered, only positions. 
% Hence, only the inter-agent potential in terms of separation distance is
% taken into consideration. 
%
% Adapted from func_swarm_2UAV_2D_decentralized.m

% 25 Apr 2011

%r0 = 2;   % desired separation

delta = pos2(1:2) - pos1(1:2);
b   = 0.1;
pos_cmd1 = zeros(4,1);
w = 0;

r = norm(delta) - r0;                 % relative distance

if abs(r) < b
    w = 0;
else if r > b
    w = (2/(1+exp(-4*(r-b)))-1)*1;          % potential, max value at r=1.5m
    else if r < -b
            w = (2/(1+exp(-4*(r+b)))-1)*1;
        end
    end
end                                       % scaled by 1.0

theta = atan2(delta(2),delta(1));

pos_cmd1(1) = w*cos(theta);
pos_cmd1(2) = w*sin(theta);

% vel_cmd2(1) = -w*cos(theta);  
% vel_cmd2(2) = -w*sin(theta);

== matlab function Agent 2/Swarming/swarm1/2 UAV Swarm Algorithm ==
  data: w output double; pos1 input double; pos_cmd1 output double; pos2 input double; r0 input double
function [w,pos_cmd1] = fcn(pos1,pos2,r0)

% Swarm algorithm for Vicon environment. 
% Heading concensus is not considered, only positions. 
% Hence, only the inter-agent potential in terms of separation distance is
% taken into consideration. 
%
% Adapted from func_swarm_2UAV_2D_decentralized.m

% 25 Apr 2011

%r0 = 2;   % desired separation

delta = pos2(1:2) - pos1(1:2);
b   = 0.1;
pos_cmd1 = zeros(4,1);
w = 0;

r = norm(delta) - r0;                 % relative distance

if abs(r) < b
    w = 0;
else if r > b
    w = (2/(1+exp(-4*(r-b)))-1)*1;          % potential, max value at r=1.5m
    else if r < -b
            w = (2/(1+exp(-4*(r+b)))-1)*1;
        end
    end
end                                       % scaled by 1.0

theta = atan2(delta(2),delta(1));

pos_cmd1(1) = w*cos(theta);
pos_cmd1(2) = w*sin(theta);

% vel_cmd2(1) = -w*cos(theta);  
% vel_cmd2(2) = -w*sin(theta);

== matlab function Agent 2/Swarming/swarm2/2 UAV Swarm Algorithm ==
  data: w output double; pos1 input double; pos_cmd1 output double; pos2 input double; r0 input double
function [w,pos_cmd1] = fcn(pos1,pos2,r0)

% Swarm algorithm for Vicon environment. 
% Heading concensus is not considered, only positions. 
% Hence, only the inter-agent potential in terms of separation distance is
% taken into consideration. 
%
% Adapted from func_swarm_2UAV_2D_decentralized.m

% 25 Apr 2011

%r0 = 2;   % desired separation

delta = pos2(1:2) - pos1(1:2);
b   = 0.1;
pos_cmd1 = zeros(4,1);
w = 0;

r = norm(delta) - r0;                 % relative distance

if abs(r) < b
    w = 0;
else if r > b
    w = (2/(1+exp(-4*(r-b)))-1)*1;          % potential, max value at r=1.5m
    else if r < -b
            w = (2/(1+exp(-4*(r+b)))-1)*1;
        end
    end
end                                       % scaled by 1.0

theta = atan2(delta(2),delta(1));

pos_cmd1(1) = w*cos(theta);
pos_cmd1(2) = w*sin(theta);

% vel_cmd2(1) = -w*cos(theta);  
% vel_cmd2(2) = -w*sin(theta);

== matlab function Agent 3/Swarming/swarm/2 UAV Swarm Algorithm ==
  data: w output double; pos1 input double; pos_cmd1 output double; pos2 input double; r0 input double
function [w,pos_cmd1] = fcn(pos1,pos2,r0)

% Swarm algorithm for Vicon environment. 
% Heading concensus is not considered, only positions. 
% Hence, only the inter-agent potential in terms of separation distance is
% taken into consideration. 
%
% Adapted from func_swarm_2UAV_2D_decentralized.m

% 25 Apr 2011

%r0 = 2;   % desired separation

delta = pos2(1:2) - pos1(1:2);
b   = 0.1;
pos_cmd1 = zeros(4,1);
w = 0;

r = norm(delta) - r0;                 % relative distance

if abs(r) < b
    w = 0;
else if r > b
    w = (2/(1+exp(-4*(r-b)))-1)*1;          % potential, max value at r=1.5m
    else if r < -b
            w = (2/(1+exp(-4*(r+b)))-1)*1;
        end
    end
end                                       % scaled by 1.0

theta = atan2(delta(2),delta(1));

pos_cmd1(1) = w*cos(theta);
pos_cmd1(2) = w*sin(theta);

% vel_cmd2(1) = -w*cos(theta);  
% vel_cmd2(2) = -w*sin(theta);

== matlab function Agent 3/Swarming/swarm1/2 UAV Swarm Algorithm ==
  data: w output double; pos1 input double; pos_cmd1 output double; pos2 input double; r0 input double
function [w,pos_cmd1] = fcn(pos1,pos2,r0)

% Swarm algorithm for Vicon environment. 
% Heading concensus is not considered, only positions. 
% Hence, only the inter-agent potential in terms of separation distance is
% taken into consideration. 
%
% Adapted from func_swarm_2UAV_2D_decentralized.m

% 25 Apr 2011

%r0 = 2;   % desired separation

delta = pos2(1:2) - pos1(1:2);
b   = 0.1;
pos_cmd1 = zeros(4,1);
w = 0;

r = norm(delta) - r0;                 % relative distance

if abs(r) < b
    w = 0;
else if r > b
    w = (2/(1+exp(-4*(r-b)))-1)*1;          % potential, max value at r=1.5m
    else if r < -b
            w = (2/(1+exp(-4*(r+b)))-1)*1;
        end
    end
end                                       % scaled by 1.0

theta = atan2(delta(2),delta(1));

pos_cmd1(1) = w*cos(theta);
pos_cmd1(2) = w*sin(theta);

% vel_cmd2(1) = -w*cos(theta);  
% vel_cmd2(2) = -w*sin(theta);

== matlab function Agent 3/Swarming/swarm2/2 UAV Swarm Algorithm ==
  data: w output double; pos1 input double; pos_cmd1 output double; pos2 input double; r0 input double
function [w,pos_cmd1] = fcn(pos1,pos2,r0)

% Swarm algorithm for Vicon environment. 
% Heading concensus is not considered, only positions. 
% Hence, only the inter-agent potential in terms of separation distance is
% taken into consideration. 
%
% Adapted from func_swarm_2UAV_2D_decentralized.m

% 25 Apr 2011

%r0 = 2;   % desired separation

delta = pos2(1:2) - pos1(1:2);
b   = 0.1;
pos_cmd1 = zeros(4,1);
w = 0;

r = norm(delta) - r0;                 % relative distance

if abs(r) < b
    w = 0;
else if r > b
    w = (2/(1+exp(-4*(r-b)))-1)*1;          % potential, max value at r=1.5m
    else if r < -b
            w = (2/(1+exp(-4*(r+b)))-1)*1;
        end
    end
end                                       % scaled by 1.0

theta = atan2(delta(2),delta(1));

pos_cmd1(1) = w*cos(theta);
pos_cmd1(2) = w*sin(theta);

% vel_cmd2(1) = -w*cos(theta);  
% vel_cmd2(2) = -w*sin(theta);

== matlab function Agent 4/Swarming/swarm/2 UAV Swarm Algorithm ==
  data: w output double; pos1 input double; pos_cmd1 output double; pos2 input double; r0 input double
function [w,pos_cmd1] = fcn(pos1,pos2,r0)

% Swarm algorithm for Vicon environment. 
% Heading concensus is not considered, only positions. 
% Hence, only the inter-agent potential in terms of separation distance is
% taken into consideration. 
%
% Adapted from func_swarm_2UAV_2D_decentralized.m

% 25 Apr 2011

%r0 = 2;   % desired separation

delta = pos2(1:2) - pos1(1:2);
b   = 0.1;
pos_cmd1 = zeros(4,1);
w = 0;

r = norm(delta) - r0;                 % relative distance

if abs(r) < b
    w = 0;
else if r > b
    w = (2/(1+exp(-4*(r-b)))-1)*1;          % potential, max value at r=1.5m
    else if r < -b
            w = (2/(1+exp(-4*(r+b)))-1)*1;
        end
    end
end                                       % scaled by 1.0

theta = atan2(delta(2),delta(1));

pos_cmd1(1) = w*cos(theta);
pos_cmd1(2) = w*sin(theta);

% vel_cmd2(1) = -w*cos(theta);  
% vel_cmd2(2) = -w*sin(theta);

== matlab function Agent 4/Swarming/swarm1/2 UAV Swarm Algorithm ==
  data: w output double; pos1 input double; pos_cmd1 output double; pos2 input double; r0 input double
function [w,pos_cmd1] = fcn(pos1,pos2,r0)

% Swarm algorithm for Vicon environment. 
% Heading concensus is not considered, only positions. 
% Hence, only the inter-agent potential in terms of separation distance is
% taken into consideration. 
%
% Adapted from func_swarm_2UAV_2D_decentralized.m

% 25 Apr 2011

%r0 = 2;   % desired separation

delta = pos2(1:2) - pos1(1:2);
b   = 0.1;
pos_cmd1 = zeros(4,1);
w = 0;

r = norm(delta) - r0;                 % relative distance

if abs(r) < b
    w = 0;
else if r > b
    w = (2/(1+exp(-4*(r-b)))-1)*1;          % potential, max value at r=1.5m
    else if r < -b
            w = (2/(1+exp(-4*(r+b)))-1)*1;
        end
    end
end                                       % scaled by 1.0

theta = atan2(delta(2),delta(1));

pos_cmd1(1) = w*cos(theta);
pos_cmd1(2) = w*sin(theta);

% vel_cmd2(1) = -w*cos(theta);  
% vel_cmd2(2) = -w*sin(theta);
